simulink model "Differential_Drive_Robot_Dynamics"  (R2017b)
settings: Solver=VariableStepAuto  StartTime=0.0  StopTime=10.0  RelTol=1e-3
settings Model: Creator=Jesus  LastModifiedBy=Jesus

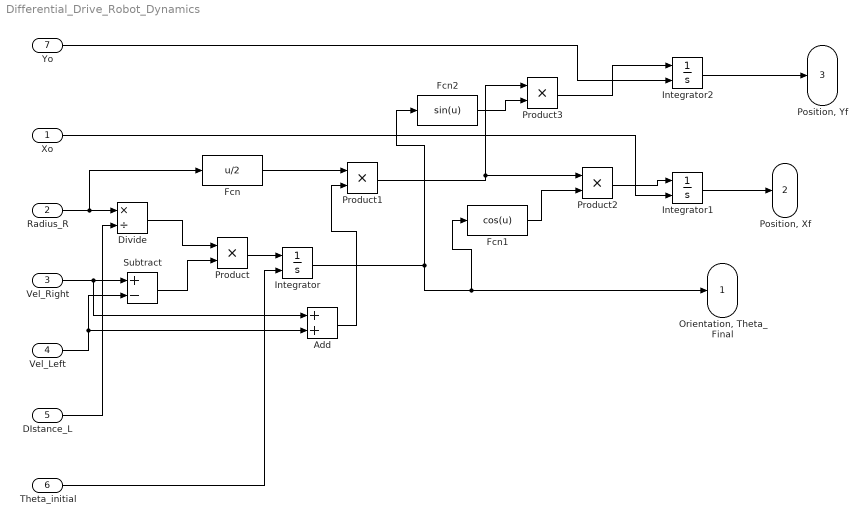
== system Differential_Drive_Robot_Dynamics ==
  Xo : Inport
  "Radius_R " : Inport  Port=2
  "Vel_Right " : Inport  Port=3
  "Vel_Left " : Inport  Port=4
  "DIstance_L " : Inport  Port=5
  " Theta_initial " : Inport  Port=6
  "Yo " : Inport  Port=7
  Add : Sum
  Divide : Product  Inputs=*/
  Fcn : Fcn  Expr=u/2
  Fcn1 : Fcn  Expr=cos(u)
  Fcn2 : Fcn  Expr=sin(u)
  Integrator : Integrator  InitialConditionSource=external
  Integrator1 : Integrator  InitialConditionSource=external
  Integrator2 : Integrator  InitialConditionSource=external
  Product{,1..3} (4 alike) : Product
  Subtract : Sum  Inputs=+-
  "Orientation, Theta_Final " : Outport
  "Position, Xf " : Outport  Port=2
  "Position, Yf" : Outport  Port=3
  wires:
  "Vel_Left "/1 -> Subtract/2, Add/2
  "Vel_Right "/1 -> Add/1, Subtract/1
  "Radius_R "/1 -> Fcn/1, Divide/1
  "DIstance_L "/1 -> Divide/2
  Subtract/1 -> Product/2
  Divide/1 -> Product/1
  Product/1 -> Integrator/1
  " Theta_initial "/1 -> Integrator/2
  Integrator/1 -> Fcn1/1, "Orientation, Theta_Final "/1, Fcn2/1
  Add/1 -> Product1/2
  Fcn/1 -> Product1/1
  Fcn1/1 -> Product2/2
  Product1/1 -> Product3/1, Product2/1
  Product2/1 -> Integrator1/1
  Xo/1 -> Integrator1/2
  Integrator1/1 -> "Position, Xf "/1
  Fcn2/1 -> Product3/2
  Product3/1 -> Integrator2/1
  "Yo "/1 -> Integrator2/2
  Integrator2/1 -> "Position, Yf"/1
